simulink model "sim_tcyb_2024_att_ctrl"  (R2020a)
settings: Solver=ode4  StartTime=0.0  StopTime=30.0  FixedStep=0.01  RelTol=1e-3
values from neighbouring files (symbols this model uses):
  c1_diff_sigma_bar_w = diag([12; 12; 12])    [init_tcyb_2024_att_ctrl.m]
  c1_diff_ui = diag([25; 30; 20])    [init_tcyb_2024_att_ctrl.m]
  c2_diff_sigma_bar_w = diag([12; 12; 12])    [init_tcyb_2024_att_ctrl.m]
  c2_diff_ui = diag([50; 50; 10])    [init_tcyb_2024_att_ctrl.m]
  c3_diff_sigma_bar_w = diag([15; 15; 15])    [init_tcyb_2024_att_ctrl.m]
  c3_diff_ui = diag([15; 15; 10])    [init_tcyb_2024_att_ctrl.m]
  dw_aa_t = 0.2 * ones(3, 5) + ( 1.0 - 0.2 ) * rand(3, 5)    [init_tcyb_2024_att_ctrl.m]
  dw_ff_t = [ 0.4 * ones(1, 5) + ( 1.0 - 0.4 ) * rand(1, 5);                      0.4 * ones(1, 5) + ( 1.0 - 0.4 ) * rand(1, 5);                      0.2 * ones(1, 5) + ( 0.6 - 0.2 ) * rand(1, 5) ]    [init_tcyb_2024_att_ctrl.m]
  dw_phi_t = ( - pi / 2 ) * ones(3, 5) + ( pi / 2 - ( - pi / 2 ) ) * rand(3, 5)    [init_tcyb_2024_att_ctrl.m]
  dwci_init = zeros(3,NF)    [init_tcyb_2024_att_ctrl.m]
  h1w = diag([20.0; 20.0; 20.0])    [init_tcyb_2024_att_ctrl.m]
  h2w = diag([30.0; 35.0; 35.0])    [init_tcyb_2024_att_ctrl.m]
  h3w = diag([30.0; 25.0; 30.0])    [init_tcyb_2024_att_ctrl.m]
  Ji = zeros(3,3,NF)    [init_tcyb_2024_att_ctrl.m]
  ksg = diag([10.0, 10.0, 8.0])    [init_tcyb_2024_att_ctrl.m]
  kw = diag([10.0, 10.0, 8.0])    [init_tcyb_2024_att_ctrl.m]
  l1 = diag([5.0, 5.0, 4.0])    [init_tcyb_2024_att_ctrl.m]
  l2 = diag([5.0, 5.0, 4.0])    [init_tcyb_2024_att_ctrl.m]
  Lamd_diff_sigma_bar_w = 0.8    [init_tcyb_2024_att_ctrl.m]
  Lamd_diff_ui = 0.8    [init_tcyb_2024_att_ctrl.m]
  mu = diag([10.0, 10.0, 10.0, 8.0, 8.0, 8.0])    [init_tcyb_2024_att_ctrl.m]
  mu_d_w = 100    [init_tcyb_2024_att_ctrl.m]
  pos0 = zeros(3, 1)    [init_tcyb_2024_att_ctrl.m]
  PZ0 = P0(3)    [init_tcyb_2024_att_ctrl.m]
  PZ1 = 10    [init_tcyb_2024_att_ctrl.m]
  R0 = 4    [init_tcyb_2024_att_ctrl.m]
  R1 = 8    [init_tcyb_2024_att_ctrl.m]
  Rei_init = zeros(3,3,NF)    [init_tcyb_2024_att_ctrl.m]
  Ri_init = zeros(3,3,NF)    [init_tcyb_2024_att_ctrl.m]
  Rx2 = 10    [init_tcyb_2024_att_ctrl.m]
  Ry2 = 6    [init_tcyb_2024_att_ctrl.m]
  Rz2 = 4    [init_tcyb_2024_att_ctrl.m]
  sgei_init = zeros(3,NF)    [init_tcyb_2024_att_ctrl.m]
  sgi_init = zeros(3,NF)    [init_tcyb_2024_att_ctrl.m]
  T0 = 0    [init_tcyb_2024_att_ctrl.m]
  T1 = tseq1    (= 10)    [init_tcyb_2024_att_ctrl.m]
  T2 = tseq1 + tseq12 + tseq2    (= 30)    [init_tcyb_2024_att_ctrl.m]
  ui_init = zeros(3,NF)    [init_tcyb_2024_att_ctrl.m]
  V_Phi_Rei_init = zeros(3,NF)    [init_tcyb_2024_att_ctrl.m]
  vel0 = zeros(3, 1)    [init_tcyb_2024_att_ctrl.m]
  wci_init = zeros(3,NF)    [init_tcyb_2024_att_ctrl.m]
  wei_init = zeros(3,NF)    [init_tcyb_2024_att_ctrl.m]
  zeta_diff_sigma_bar_w = 0.3    [init_tcyb_2024_att_ctrl.m]
  zeta_diff_ui = 0.05    [init_tcyb_2024_att_ctrl.m]
undefined symbols (not defined in the file or in its folder): cal_frac_squ, p_alfaw1, p_alfaw2, q_alfaw1, q_alfaw2, wi_init
(part 4 of 5)

== matlab function sim_tcyb_2024_att_ctrl/combine wei Qei Rei ==
  data: wei_1 input; wei_vec output; wei_2 input; wei_3 input; wei_4 input; wei_5 input; sgei_1 input; sgei_2 input; sgei_3 input; sgei_4 input; sgei_5 input; Rei_1 input; Rei_2 input; Rei_3 input; Rei_4 input; Rei_5 input; sgei_vec output; Rei_vec output
function [wei_vec, sgei_vec, Rei_vec] = fcn(wei_1, wei_2, wei_3, wei_4, wei_5, ...
                                                                                sgei_1, sgei_2, sgei_3, sgei_4, sgei_5, ...
                                                                                Rei_1, Rei_2, Rei_3, Rei_4, Rei_5)
%%%% 合并姿态角速率误差/四元数误差/姿态旋转矩阵误差
wei_vec = zeros(3,5);
wei_vec(:,1) = wei_1(:);
wei_vec(:,2) = wei_2(:);
wei_vec(:,3) = wei_3(:);
wei_vec(:,4) = wei_4(:);
wei_vec(:,5) = wei_5(:);

sgei_vec = zeros(3,5);
sgei_vec(:,1) = sgei_1(:);
sgei_vec(:,2) = sgei_2(:);
sgei_vec(:,3) = sgei_3(:);
sgei_vec(:,4) = sgei_4(:);
sgei_vec(:,5) = sgei_5(:);

Rei_vec = zeros(3,3,5);
Rei_vec(:,:,1) = Rei_1;
Rei_vec(:,:,2) = Rei_2;
Rei_vec(:,:,3) = Rei_3;
Rei_vec(:,:,4) = Rei_4;
Rei_vec(:,:,5) = Rei_5;

== matlab function sim_tcyb_2024_att_ctrl/cal Ri agent 1 ==
  data: Ri_1 output; sgi_vec input
function Ri_1 = fcn(sgi_vec)
%%%% 由罗德里格常量sgi求解姿态旋转矩阵Ri
iiuav = 1;
Ri_1 = eye(3) + 4 * ( 1 - ( ( ( sgi_vec(:,iiuav)' ) * sgi_vec(:,iiuav) ) / ( ( 1 + ( sgi_vec(:,iiuav)' ) * sgi_vec(:,iiuav) ) ^ 2 ) ) ) * cal_askew_mat( sgi_vec(:,iiuav) ) ...
                            + ( 8 / ( ( 1 + ( sgi_vec(:,iiuav)' ) * sgi_vec(:,iiuav) ) ^ 2 ) ) * cal_askew_mat( sgi_vec(:,iiuav) ) * cal_askew_mat( sgi_vec(:,iiuav) );
Ri_1 = Ri_1';
end

== matlab function sim_tcyb_2024_att_ctrl/combine E_sgi_vec ==
  data: E_sgi_1 input; E_sgi_vec output; E_sgi_2 input; E_sgi_3 input; E_sgi_4 input; E_sgi_5 input
function E_sgi_vec = fcn(E_sgi_1, E_sgi_2, E_sgi_3, E_sgi_4, E_sgi_5)
%%%% 合并姿态计算矩阵
E_sgi_vec = zeros(3,3,5);
E_sgi_vec(:,:,1) = E_sgi_1;
E_sgi_vec(:,:,2) = E_sgi_2;
E_sgi_vec(:,:,3) = E_sgi_3;
E_sgi_vec(:,:,4) = E_sgi_4;
E_sgi_vec(:,:,5) = E_sgi_5;

== matlab function sim_tcyb_2024_att_ctrl/cal differentiator d_sigma_bar_w_hat agent 3/choose sigma_bar_w ==
  data: x input; y output
function y = fcn(x)
iiuav = 3;
y = x(:,iiuav);

== matlab function sim_tcyb_2024_att_ctrl/cal differentiator d_sigma_bar_w_hat agent 3/trans to column20 ==
  data: x input; y output
function y = fcn(x)
y = x(:);

== matlab function sim_tcyb_2024_att_ctrl/cal differentiator d_sigma_bar_w_hat agent 3/trans to column21 ==
  data: x input; y output
function y = fcn(x)
y = x(:);

== matlab function sim_tcyb_2024_att_ctrl/cal differentiator d_sigma_bar_w_hat agent 3/trans to column22 ==
  data: x input; y output
function y = fcn(x)
y = x(:);

== matlab function sim_tcyb_2024_att_ctrl/cal differentiator d_sigma_bar_w_hat agent 3/trans to column23 ==
  data: x input; y output
function y = fcn(x)
y = x(:);

== matlab function sim_tcyb_2024_att_ctrl/combine Qci Rci1 ==
  data: V_Phi_Rei_1 input; V_Phi_Rei_vec output; V_Phi_Rei_2 input; V_Phi_Rei_3 input; V_Phi_Rei_4 input; V_Phi_Rei_5 input
function V_Phi_Rei_vec = fcn(V_Phi_Rei_1, V_Phi_Rei_2, V_Phi_Rei_3, V_Phi_Rei_4, V_Phi_Rei_5)
%%%% 合并LogSO3空间的辅助姿态误差向量
V_Phi_Rei_vec = [V_Phi_Rei_1(:), V_Phi_Rei_2(:), V_Phi_Rei_3(:), V_Phi_Rei_4(:), V_Phi_Rei_5(:)];

== matlab function sim_tcyb_2024_att_ctrl/depart sge1 ==
  data: y output; x input
function y = fcn(x)
y = x(:,1);

end

== matlab function sim_tcyb_2024_att_ctrl/depart sge2 ==
  data: y output; x input
function y = fcn(x)
y = x(:,2);

end

== matlab function sim_tcyb_2024_att_ctrl/depart sge3 ==
  data: y output; x input
function y = fcn(x)
y = x(:,3);

end

== matlab function sim_tcyb_2024_att_ctrl/depart sge4 ==
  data: y output; x input
function y = fcn(x)
y = x(:,4);

end

== matlab function sim_tcyb_2024_att_ctrl/depart sge5 ==
  data: y output; x input
function y = fcn(x)
y = x(:,5);

end

== matlab function sim_tcyb_2024_att_ctrl/depart we1 ==
  data: y output; x input
function y = fcn(x)
y = x(:,1);

end

== matlab function sim_tcyb_2024_att_ctrl/depart we2 ==
  data: y output; x input
function y = fcn(x)
y = x(:,2);

end

== matlab function sim_tcyb_2024_att_ctrl/depart we3 ==
  data: y output; x input
function y = fcn(x)
y = x(:,3);

end

== matlab function sim_tcyb_2024_att_ctrl/depart we4 ==
  data: y output; x input
function y = fcn(x)
y = x(:,4);

end

== matlab function sim_tcyb_2024_att_ctrl/E_sgi agent 3 ==
  data: sgi_vec input; E_sgi_3 output
function E_sgi_3 = fcn(sgi_vec)
%%%% 更新四元数微分方程
iiuav = 3;
E_sgi_3 = (1/4) * ( ( 1 - (sgi_vec(:,iiuav)') * sgi_vec(:,iiuav) ) * eye(3) ...
                    + 2 * cal_askew_mat( sgi_vec(:,iiuav) ) + 2 * sgi_vec(:,iiuav) * ( sgi_vec(:,iiuav)' ) );
end

== matlab function sim_tcyb_2024_att_ctrl/depart we5 ==
  data: y output; x input
function y = fcn(x)
y = x(:,5);

end

== matlab function sim_tcyb_2024_att_ctrl/depart V_Phi_Re5 ==
  data: y output; x input
function y = fcn(x)
y = x(:,5);

end

== matlab function sim_tcyb_2024_att_ctrl/depart V_Phi_Re1 ==
  data: y output; x input
function y = fcn(x)
y = x(:,1);

end

== matlab function sim_tcyb_2024_att_ctrl/depart V_Phi_Re2 ==
  data: y output; x input
function y = fcn(x)
y = x(:,2);

end

== matlab function sim_tcyb_2024_att_ctrl/depart V_Phi_Re3 ==
  data: y output; x input
function y = fcn(x)
y = x(:,3);

end

== matlab function sim_tcyb_2024_att_ctrl/depart V_Phi_Re4 ==
  data: y output; x input
function y = fcn(x)
y = x(:,4);

end

== matlab function sim_tcyb_2024_att_ctrl/cal differentiator d_sigma_bar_w_hat agent 3/trans to column24 ==
  data: x input; y output
function y = fcn(x)
y = x(:);

== matlab function sim_tcyb_2024_att_ctrl/cal differentiator d_sigma_bar_w_hat agent 3/trans to column25 ==
  data: x input; y output
function y = fcn(x)
y = x(:);

== matlab function sim_tcyb_2024_att_ctrl/cal differentiator d_sigma_bar_w_hat agent 4/cal differentiator ==
  data: c1 input; d_sigma_bar_v_hat output; d_dsigma_bar_v_hat output; d_d2sigma_bar_v_hat output; c2 input; c3 input; chi_t input; sigma_bar_v_sig_1 input; sigma_bar_v_sig_2 input; sigma_bar_v_sig_3 input; sigma_bar_v_sig_4 input; sigma_bar_v_sig_5 input; sigma_bar_v_sig_6 input; d_sigma_bar_v_hat input; d2_sigma_bar_v_hat input
function [d_sigma_bar_v_hat, d_dsigma_bar_v_hat, d_d2sigma_bar_v_hat] = fcn(c1, c2, c3, chi_t, sigma_bar_v_sig_1, sigma_bar_v_sig_2, sigma_bar_v_sig_3, ...
                                                                                                                                                sigma_bar_v_sig_4, sigma_bar_v_sig_5, sigma_bar_v_sig_6, d_sigma_bar_v_hat, d2_sigma_bar_v_hat)
d_d2sigma_bar_v_hat = -chi_t .* c1 * sigma_bar_v_sig_1(:) - (1 - chi_t) .* c1 * sigma_bar_v_sig_2(:);
d_dsigma_bar_v_hat = -chi_t .* c2 * sigma_bar_v_sig_3(:) - (1 - chi_t) .* c2 * sigma_bar_v_sig_4(:) + d2_sigma_bar_v_hat(:);
d_sigma_bar_v_hat = -chi_t .* c3 * sigma_bar_v_sig_5(:) - (1 - chi_t) .* c3 * sigma_bar_v_sig_6(:) + d_sigma_bar_v_hat(:);

== matlab function sim_tcyb_2024_att_ctrl/sgi dynam agent 3 ==
  data: E_sgi_vec input; dsgi_3 output; wi_vec input
function dsgi_3 = fcn(E_sgi_vec, wi_vec)
%%%% 更新四元数微分方程
iiuav = 3;
dsgi_3 = E_sgi_vec(:,:,iiuav) * wi_vec(:,iiuav);
end

== matlab function sim_tcyb_2024_att_ctrl/cal differentiator d_sigma_bar_w_hat agent 4/cal sig ==
  data: x input; z output; y input
function z = fcn(x, y)
z = x(:) .* sign(y(:));

== matlab function sim_tcyb_2024_att_ctrl/cal differentiator d_sigma_bar_w_hat agent 4/cal sig1 ==
  data: x input; z output; y input
function z = fcn(x, y)
z = x(:) .* sign(y(:));

== matlab function sim_tcyb_2024_att_ctrl/cal differentiator d_sigma_bar_w_hat agent 4/cal sig2 ==
  data: x input; z output; y input
function z = fcn(x, y)
z = x(:) .* sign(y(:));

== matlab function sim_tcyb_2024_att_ctrl/cal differentiator d_sigma_bar_w_hat agent 4/cal sig3 ==
  data: x input; z output; y input
function z = fcn(x, y)
z = x(:) .* sign(y(:));

== matlab function sim_tcyb_2024_att_ctrl/cal differentiator d_sigma_bar_w_hat agent 4/cal sig4 ==
  data: x input; z output; y input
function z = fcn(x, y)
z = x(:) .* sign(y(:));

== matlab function sim_tcyb_2024_att_ctrl/cal differentiator d_sigma_bar_w_hat agent 4/cal sig5 ==
  data: x input; z output; y input
function z = fcn(x, y)
z = x(:) .* sign(y(:));

== matlab function sim_tcyb_2024_att_ctrl/cal differentiator d_sigma_bar_w_hat agent 4/choose sigma_bar_w ==
  data: x input; y output
function y = fcn(x)
iiuav = 4;
y = x(:,iiuav);

== matlab function sim_tcyb_2024_att_ctrl/cal differentiator d_sigma_bar_w_hat agent 4/trans to column20 ==
  data: x input; y output
function y = fcn(x)
y = x(:);

== matlab function sim_tcyb_2024_att_ctrl/cal differentiator d_sigma_bar_w_hat agent 4/trans to column21 ==
  data: x input; y output
function y = fcn(x)
y = x(:);

== matlab function sim_tcyb_2024_att_ctrl/cal differentiator d_sigma_bar_w_hat agent 4/trans to column22 ==
  data: x input; y output
function y = fcn(x)
y = x(:);

== matlab function sim_tcyb_2024_att_ctrl/cal Ri agent 4 ==
  data: Ri_4 output; sgi_vec input
function Ri_4 = fcn(sgi_vec)
%%%% 由罗德里格常量sgi求解姿态旋转矩阵Ri
iiuav = 4;
Ri_4 = eye(3) + 4 * ( 1 - ( ( ( sgi_vec(:,iiuav)' ) * sgi_vec(:,iiuav) ) / ( ( 1 + ( sgi_vec(:,iiuav)' ) * sgi_vec(:,iiuav) ) ^ 2 ) ) ) * cal_askew_mat( sgi_vec(:,iiuav) ) ...
                            + ( 8 / ( ( 1 + ( sgi_vec(:,iiuav)' ) * sgi_vec(:,iiuav) ) ^ 2 ) ) * cal_askew_mat( sgi_vec(:,iiuav) ) * cal_askew_mat( sgi_vec(:,iiuav) );
Ri_4 = Ri_4';
end

== matlab function sim_tcyb_2024_att_ctrl/cal differentiator d_sigma_bar_w_hat agent 4/trans to column23 ==
  data: x input; y output
function y = fcn(x)
y = x(:);

== matlab function sim_tcyb_2024_att_ctrl/cal differentiator d_sigma_bar_w_hat agent 4/trans to column24 ==
  data: x input; y output
function y = fcn(x)
y = x(:);

== matlab function sim_tcyb_2024_att_ctrl/cal differentiator d_sigma_bar_w_hat agent 4/trans to column25 ==
  data: x input; y output
function y = fcn(x)
y = x(:);

== matlab function sim_tcyb_2024_att_ctrl/cal differentiator d_sigma_bar_w_hat agent 5/cal differentiator ==
  data: c1 input; d_sigma_bar_v_hat output; d_dsigma_bar_v_hat output; d_d2sigma_bar_v_hat output; c2 input; c3 input; chi_t input; sigma_bar_v_sig_1 input; sigma_bar_v_sig_2 input; sigma_bar_v_sig_3 input; sigma_bar_v_sig_4 input; sigma_bar_v_sig_5 input; sigma_bar_v_sig_6 input; d_sigma_bar_v_hat input; d2_sigma_bar_v_hat input
function [d_sigma_bar_v_hat, d_dsigma_bar_v_hat, d_d2sigma_bar_v_hat] = fcn(c1, c2, c3, chi_t, sigma_bar_v_sig_1, sigma_bar_v_sig_2, sigma_bar_v_sig_3, ...
                                                                                                                                                sigma_bar_v_sig_4, sigma_bar_v_sig_5, sigma_bar_v_sig_6, d_sigma_bar_v_hat, d2_sigma_bar_v_hat)
d_d2sigma_bar_v_hat = -chi_t .* c1 * sigma_bar_v_sig_1(:) - (1 - chi_t) .* c1 * sigma_bar_v_sig_2(:);
d_dsigma_bar_v_hat = -chi_t .* c2 * sigma_bar_v_sig_3(:) - (1 - chi_t) .* c2 * sigma_bar_v_sig_4(:) + d2_sigma_bar_v_hat(:);
d_sigma_bar_v_hat = -chi_t .* c3 * sigma_bar_v_sig_5(:) - (1 - chi_t) .* c3 * sigma_bar_v_sig_6(:) + d_sigma_bar_v_hat(:);

== matlab function sim_tcyb_2024_att_ctrl/cal differentiator d_sigma_bar_w_hat agent 5/cal sig ==
  data: x input; z output; y input
function z = fcn(x, y)
z = x(:) .* sign(y(:));

== matlab function sim_tcyb_2024_att_ctrl/cal differentiator d_sigma_bar_w_hat agent 5/cal sig1 ==
  data: x input; z output; y input
function z = fcn(x, y)
z = x(:) .* sign(y(:));

== matlab function sim_tcyb_2024_att_ctrl/cal differentiator d_sigma_bar_w_hat agent 5/cal sig2 ==
  data: x input; z output; y input
function z = fcn(x, y)
z = x(:) .* sign(y(:));

== matlab function sim_tcyb_2024_att_ctrl/E_sgi agent 4 ==
  data: sgi_vec input; E_sgi_4 output
function E_sgi_4 = fcn(sgi_vec)
%%%% 更新四元数微分方程
iiuav = 4;
E_sgi_4 = (1/4) * ( ( 1 - (sgi_vec(:,iiuav)') * sgi_vec(:,iiuav) ) * eye(3) ...
                    + 2 * cal_askew_mat( sgi_vec(:,iiuav) ) + 2 * sgi_vec(:,iiuav) * ( sgi_vec(:,iiuav)' ) );
end

== matlab function sim_tcyb_2024_att_ctrl/cal differentiator d_sigma_bar_w_hat agent 5/cal sig3 ==
  data: x input; z output; y input
function z = fcn(x, y)
z = x(:) .* sign(y(:));

== matlab function sim_tcyb_2024_att_ctrl/cal differentiator d_sigma_bar_w_hat agent 5/cal sig4 ==
  data: x input; z output; y input
function z = fcn(x, y)
z = x(:) .* sign(y(:));

== matlab function sim_tcyb_2024_att_ctrl/cal differentiator d_sigma_bar_w_hat agent 5/cal sig5 ==
  data: x input; z output; y input
function z = fcn(x, y)
z = x(:) .* sign(y(:));

== matlab function sim_tcyb_2024_att_ctrl/cal differentiator d_sigma_bar_w_hat agent 5/choose sigma_bar_w ==
  data: x input; y output
function y = fcn(x)
iiuav = 5;
y = x(:,iiuav);

== matlab function sim_tcyb_2024_att_ctrl/cal differentiator d_sigma_bar_w_hat agent 5/trans to column20 ==
  data: x input; y output
function y = fcn(x)
y = x(:);

== matlab function sim_tcyb_2024_att_ctrl/cal differentiator d_sigma_bar_w_hat agent 5/trans to column21 ==
  data: x input; y output
function y = fcn(x)
y = x(:);

== matlab function sim_tcyb_2024_att_ctrl/cal differentiator d_sigma_bar_w_hat agent 5/trans to column22 ==
  data: x input; y output
function y = fcn(x)
y = x(:);

== matlab function sim_tcyb_2024_att_ctrl/cal differentiator d_sigma_bar_w_hat agent 5/trans to column23 ==
  data: x input; y output
function y = fcn(x)
y = x(:);

== matlab function sim_tcyb_2024_att_ctrl/cal differentiator d_sigma_bar_w_hat agent 5/trans to column24 ==
  data: x input; y output
function y = fcn(x)
y = x(:);

== matlab function sim_tcyb_2024_att_ctrl/cal differentiator d_sigma_bar_w_hat agent 5/trans to column25 ==
  data: x input; y output
function y = fcn(x)
y = x(:);

== matlab function sim_tcyb_2024_att_ctrl/sgi dynam agent 4 ==
  data: E_sgi_vec input; dsgi_4 output; wi_vec input
function dsgi_4 = fcn(E_sgi_vec, wi_vec)
%%%% 更新四元数微分方程
iiuav = 4;
dsgi_4 = E_sgi_vec(:,:,iiuav) * wi_vec(:,iiuav);
end

== matlab function sim_tcyb_2024_att_ctrl/cal dw_hat agent 1 ==
  data: h3w input; Ji input; d_sigma_bar_w_vec input; sigma_bar_w_hat_vec input; dw_hat_1 output
function dw_hat_1 = fcn(h3w, Ji, d_sigma_bar_w_vec, sigma_bar_w_hat_vec)
%%%% 计算扰动观测值dw_hat
iiuav = 1;
dw_hat_1 = Ji(:,:,iiuav) * d_sigma_bar_w_vec(:,iiuav) + h3w * sigma_bar_w_hat_vec(:,iiuav);

== matlab function sim_tcyb_2024_att_ctrl/cal dw_hat agent 2 ==
  data: h3w input; Ji input; d_sigma_bar_w_vec input; sigma_bar_w_hat_vec input; dw_hat_2 output
function dw_hat_2 = fcn(h3w, Ji, d_sigma_bar_w_vec, sigma_bar_w_hat_vec)
%%%% 计算扰动观测值dw_hat
iiuav = 2;
dw_hat_2 = Ji(:,:,iiuav) * d_sigma_bar_w_vec(:,iiuav) + h3w * sigma_bar_w_hat_vec(:,iiuav);

== matlab function sim_tcyb_2024_att_ctrl/cal dw_hat agent 3 ==
  data: h3w input; Ji input; d_sigma_bar_w_vec input; sigma_bar_w_hat_vec input; dw_hat_3 output
function dw_hat_3 = fcn(h3w, Ji, d_sigma_bar_w_vec, sigma_bar_w_hat_vec)
%%%% 计算扰动观测值dw_hat
iiuav = 3;
dw_hat_3 = Ji(:,:,iiuav) * d_sigma_bar_w_vec(:,iiuav) + h3w * sigma_bar_w_hat_vec(:,iiuav);

== matlab function sim_tcyb_2024_att_ctrl/cal dw_hat agent 4 ==
  data: h3w input; Ji input; d_sigma_bar_w_vec input; sigma_bar_w_hat_vec input; dw_hat_4 output
function dw_hat_4 = fcn(h3w, Ji, d_sigma_bar_w_vec, sigma_bar_w_hat_vec)
%%%% 计算扰动观测值dw_hat
iiuav = 4;
dw_hat_4 = Ji(:,:,iiuav) * d_sigma_bar_w_vec(:,iiuav) + h3w * sigma_bar_w_hat_vec(:,iiuav);

== matlab function sim_tcyb_2024_att_ctrl/cal dw_hat agent 5 ==
  data: h3w input; Ji input; d_sigma_bar_w_vec input; sigma_bar_w_hat_vec input; dw_hat_5 output
function dw_hat_5 = fcn(h3w, Ji, d_sigma_bar_w_vec, sigma_bar_w_hat_vec)
%%%% 计算扰动观测值dw_hat
iiuav = 5;
dw_hat_5 = Ji(:,:,iiuav) * d_sigma_bar_w_vec(:,iiuav) + h3w * sigma_bar_w_hat_vec(:,iiuav);

== matlab function sim_tcyb_2024_att_ctrl/cal error dw_tilt ==
  data: dw_vec input; dw_hat_vec input; dw_tilt_vec output
function dw_tilt_vec = fcn(dw_vec, dw_hat_vec)
%%%% 计算扰动观测误差dw_tilt
dw_tilt_vec = zeros(3,5);
for iiuav = 1:5
    dw_tilt_vec(:,iiuav) = dw_vec(:,iiuav) - dw_hat_vec(:,iiuav);
end

== matlab function sim_tcyb_2024_att_ctrl/cal sigma_bar_w_hat agent 1 ==
  data: h1w input; h2w input; theta_sigma_bar_w_tilt_1_vec input; d_sigma_bar_w_hat_1 output; theta_sigma_bar_w_tilt_2_vec input; d_sigma_bar_w_vec input
function d_sigma_bar_w_hat_1 = fcn(h1w, h2w, theta_sigma_bar_w_tilt_1_vec, theta_sigma_bar_w_tilt_2_vec, d_sigma_bar_w_vec)
%%%% 计算扰动观测器中虚拟速度控制量观测值sigma_w_hat的微分方程
iiuav = 1;
d_sigma_bar_w_hat_1 = d_sigma_bar_w_vec(:,iiuav) + ...
                                            h1w * theta_sigma_bar_w_tilt_1_vec(:,iiuav) + ...
                                            h2w * theta_sigma_bar_w_tilt_2_vec(:,iiuav);

== matlab function sim_tcyb_2024_att_ctrl/cal sigma_bar_w_hat agent 2 ==
  data: h1w input; h2w input; theta_sigma_bar_w_tilt_1_vec input; d_sigma_bar_w_hat_2 output; theta_sigma_bar_w_tilt_2_vec input; d_sigma_bar_w_vec input
function d_sigma_bar_w_hat_2 = fcn(h1w, h2w, theta_sigma_bar_w_tilt_1_vec, theta_sigma_bar_w_tilt_2_vec, d_sigma_bar_w_vec)
%%%% 计算扰动观测器中虚拟速度控制量观测值sigma_v_hat的微分方程
iiuav = 2;
d_sigma_bar_w_hat_2 = d_sigma_bar_w_vec(:,iiuav) + ...
                                            h1w * theta_sigma_bar_w_tilt_1_vec(:,iiuav) + ...
                                            h2w * theta_sigma_bar_w_tilt_2_vec(:,iiuav);

== matlab function sim_tcyb_2024_att_ctrl/cal Ri agent 5 ==
  data: Ri_5 output; sgi_vec input
function Ri_5 = fcn(sgi_vec)
%%%% 由罗德里格常量sgi求解姿态旋转矩阵Ri
iiuav = 5;
Ri_5 = eye(3) + 4 * ( 1 - ( ( ( sgi_vec(:,iiuav)' ) * sgi_vec(:,iiuav) ) / ( ( 1 + ( sgi_vec(:,iiuav)' ) * sgi_vec(:,iiuav) ) ^ 2 ) ) ) * cal_askew_mat( sgi_vec(:,iiuav) ) ...
                            + ( 8 / ( ( 1 + ( sgi_vec(:,iiuav)' ) * sgi_vec(:,iiuav) ) ^ 2 ) ) * cal_askew_mat( sgi_vec(:,iiuav) ) * cal_askew_mat( sgi_vec(:,iiuav) );
Ri_5 = Ri_5';
end

== matlab function sim_tcyb_2024_att_ctrl/cal sigma_bar_w_hat agent 3 ==
  data: h1w input; h2w input; theta_sigma_bar_w_tilt_1_vec input; d_sigma_bar_w_hat_3 output; theta_sigma_bar_w_tilt_2_vec input; d_sigma_bar_w_vec input
function d_sigma_bar_w_hat_3 = fcn(h1w, h2w, theta_sigma_bar_w_tilt_1_vec, theta_sigma_bar_w_tilt_2_vec, d_sigma_bar_w_vec)
%%%% 计算扰动观测器中虚拟速度控制量观测值sigma_w_hat的微分方程
iiuav = 3;
d_sigma_bar_w_hat_3 = d_sigma_bar_w_vec(:,iiuav) + ...
                                            h1w * theta_sigma_bar_w_tilt_1_vec(:,iiuav) + ...
                                            h2w * theta_sigma_bar_w_tilt_2_vec(:,iiuav);

== matlab function sim_tcyb_2024_att_ctrl/cal sigma_bar_w_hat agent 4 ==
  data: h1w input; h2w input; theta_sigma_bar_w_tilt_1_vec input; d_sigma_bar_w_hat_4 output; theta_sigma_bar_w_tilt_2_vec input; d_sigma_bar_w_vec input
function d_sigma_bar_w_hat_4 = fcn(h1w, h2w, theta_sigma_bar_w_tilt_1_vec, theta_sigma_bar_w_tilt_2_vec, d_sigma_bar_w_vec)
%%%% 计算扰动观测器中虚拟速度控制量观测值sigma_w_hat的微分方程
iiuav = 4;
d_sigma_bar_w_hat_4 = d_sigma_bar_w_vec(:,iiuav) + ...
                                            h1w * theta_sigma_bar_w_tilt_1_vec(:,iiuav) + ...
                                            h2w * theta_sigma_bar_w_tilt_2_vec(:,iiuav);

== matlab function sim_tcyb_2024_att_ctrl/cal sigma_bar_w_hat agent 5 ==
  data: h1w input; h2w input; theta_sigma_bar_w_tilt_1_vec input; d_sigma_bar_w_hat_5 output; theta_sigma_bar_w_tilt_2_vec input; d_sigma_bar_w_vec input
function d_sigma_bar_w_hat_5 = fcn(h1w, h2w, theta_sigma_bar_w_tilt_1_vec, theta_sigma_bar_w_tilt_2_vec, d_sigma_bar_w_vec)
%%%% 计算扰动观测器中虚拟速度控制量观测值sigma_w_hat的微分方程
iiuav = 5;
d_sigma_bar_w_hat_5 = d_sigma_bar_w_vec(:,iiuav) + ...
                                            h1w * theta_sigma_bar_w_tilt_1_vec(:,iiuav) + ...
                                            h2w * theta_sigma_bar_w_tilt_2_vec(:,iiuav);

== matlab function sim_tcyb_2024_att_ctrl/cal sigma_w_bar ==
  data: sigma_bar_w_vec output; wi_vec input; sigma_w_vec input
function sigma_bar_w_vec = fcn(wi_vec, sigma_w_vec)
%%%% 计算姿态角速率跟踪误差
sigma_bar_w_vec = zeros(3,5);
for iiuav = 1:5
    sigma_bar_w_vec(:,iiuav) = wi_vec(:,iiuav) - sigma_w_vec(:,iiuav);
end

== matlab function sim_tcyb_2024_att_ctrl/cal theta_sigma_bar_w_tilt agent 1 ==
  data: alfa_theta_obs_w input; sigma_bar_w_tilt_squ_1_1 input; theta_sigma_bar_w_tilt_1_1 output; sigma_bar_w_tilt_squ_2_1 input; sigma_bar_w_tilt_vec input; theta_sigma_bar_w_tilt_2_1 output
function [theta_sigma_bar_w_tilt_1_1, theta_sigma_bar_w_tilt_2_1] = fcn(alfa_theta_obs_w, sigma_bar_w_tilt_squ_1_1, sigma_bar_w_tilt_squ_2_1, sigma_bar_w_tilt_vec)
%%%% 计算平滑递增函数
iiuav = 1;
theta_sigma_bar_w_tilt_1_1 = sigma_bar_w_tilt_squ_1_1(:) .* ( -1 + 2 ./ ( 1 + exp( -alfa_theta_obs_w .* sigma_bar_w_tilt_vec(:,iiuav) ) ) );
theta_sigma_bar_w_tilt_2_1 = sigma_bar_w_tilt_squ_2_1(:) .* ( -1 + 2 ./ ( 1 + exp( -alfa_theta_obs_w .* sigma_bar_w_tilt_vec(:,iiuav) ) ) );

== matlab function sim_tcyb_2024_att_ctrl/cal theta_sigma_bar_w_tilt agent 2 ==
  data: alfa_theta_obs_w input; sigma_bar_w_tilt_squ_1_2 input; theta_sigma_bar_w_tilt_1_2 output; sigma_bar_w_tilt_squ_2_2 input; sigma_bar_w_tilt_vec input; theta_sigma_bar_w_tilt_2_2 output
function [theta_sigma_bar_w_tilt_1_2, theta_sigma_bar_w_tilt_2_2] = fcn(alfa_theta_obs_w, sigma_bar_w_tilt_squ_1_2, sigma_bar_w_tilt_squ_2_2, sigma_bar_w_tilt_vec)
%%%% 计算平滑递增函数
iiuav = 2;
theta_sigma_bar_w_tilt_1_2 = sigma_bar_w_tilt_squ_1_2(:) .* ( -1 + 2 ./ ( 1 + exp( -alfa_theta_obs_w .* sigma_bar_w_tilt_vec(:,iiuav) ) ) );
theta_sigma_bar_w_tilt_2_2 = sigma_bar_w_tilt_squ_2_2(:) .* ( -1 + 2 ./ ( 1 + exp( -alfa_theta_obs_w .* sigma_bar_w_tilt_vec(:,iiuav) ) ) );

== matlab function sim_tcyb_2024_att_ctrl/cal theta_sigma_bar_w_tilt agent 3 ==
  data: alfa_theta_obs_w input; sigma_bar_w_tilt_squ_1_3 input; theta_sigma_bar_w_tilt_1_3 output; sigma_bar_w_tilt_squ_2_3 input; sigma_bar_w_tilt_vec input; theta_sigma_bar_w_tilt_2_3 output
function [theta_sigma_bar_w_tilt_1_3, theta_sigma_bar_w_tilt_2_3] = fcn(alfa_theta_obs_w, sigma_bar_w_tilt_squ_1_3, sigma_bar_w_tilt_squ_2_3, sigma_bar_w_tilt_vec)
%%%% 计算平滑递增函数
iiuav = 3;
theta_sigma_bar_w_tilt_1_3 = sigma_bar_w_tilt_squ_1_3(:) .* ( -1 + 2 ./ ( 1 + exp( -alfa_theta_obs_w .* sigma_bar_w_tilt_vec(:,iiuav) ) ) );
theta_sigma_bar_w_tilt_2_3 = sigma_bar_w_tilt_squ_2_3(:) .* ( -1 + 2 ./ ( 1 + exp( -alfa_theta_obs_w .* sigma_bar_w_tilt_vec(:,iiuav) ) ) );

== matlab function sim_tcyb_2024_att_ctrl/E_sgi agent 5 ==
  data: sgi_vec input; E_sgi_5 output
function E_sgi_5 = fcn(sgi_vec)
%%%% 更新四元数微分方程
iiuav = 5;
E_sgi_5 = (1/4) * ( ( 1 - (sgi_vec(:,iiuav)') * sgi_vec(:,iiuav) ) * eye(3) ...
                    + 2 * cal_askew_mat( sgi_vec(:,iiuav) ) + 2 * sgi_vec(:,iiuav) * ( sgi_vec(:,iiuav)' ) );
end

== matlab function sim_tcyb_2024_att_ctrl/cal theta_sigma_bar_w_tilt agent 4 ==
  data: alfa_theta_obs_w input; sigma_bar_w_tilt_squ_1_4 input; theta_sigma_bar_w_tilt_1_4 output; sigma_bar_w_tilt_squ_2_4 input; sigma_bar_w_tilt_vec input; theta_sigma_bar_w_tilt_2_4 output
function [theta_sigma_bar_w_tilt_1_4, theta_sigma_bar_w_tilt_2_4] = fcn(alfa_theta_obs_w, sigma_bar_w_tilt_squ_1_4, sigma_bar_w_tilt_squ_2_4, sigma_bar_w_tilt_vec)
%%%% 计算平滑递增函数
iiuav = 4;
theta_sigma_bar_w_tilt_1_4 = sigma_bar_w_tilt_squ_1_4(:) .* ( -1 + 2 ./ ( 1 + exp( -alfa_theta_obs_w .* sigma_bar_w_tilt_vec(:,iiuav) ) ) );
theta_sigma_bar_w_tilt_2_4 = sigma_bar_w_tilt_squ_2_4(:) .* ( -1 + 2 ./ ( 1 + exp( -alfa_theta_obs_w .* sigma_bar_w_tilt_vec(:,iiuav) ) ) );

== matlab function sim_tcyb_2024_att_ctrl/cal theta_sigma_bar_w_tilt agent 5 ==
  data: alfa_theta_obs_w input; sigma_bar_w_tilt_squ_1_5 input; theta_sigma_bar_w_tilt_1_5 output; sigma_bar_w_tilt_squ_2_5 input; sigma_bar_w_tilt_vec input; theta_sigma_bar_w_tilt_2_5 output
function [theta_sigma_bar_w_tilt_1_5, theta_sigma_bar_w_tilt_2_5] = fcn(alfa_theta_obs_w, sigma_bar_w_tilt_squ_1_5, sigma_bar_w_tilt_squ_2_5, sigma_bar_w_tilt_vec)
%%%% 计算平滑递增函数
iiuav = 5;
theta_sigma_bar_w_tilt_1_5 = sigma_bar_w_tilt_squ_1_5(:) .* ( -1 + 2 ./ ( 1 + exp( -alfa_theta_obs_w .* sigma_bar_w_tilt_vec(:,iiuav) ) ) );
theta_sigma_bar_w_tilt_2_5 = sigma_bar_w_tilt_squ_2_5(:) .* ( -1 + 2 ./ ( 1 + exp( -alfa_theta_obs_w .* sigma_bar_w_tilt_vec(:,iiuav) ) ) );

== matlab function sim_tcyb_2024_att_ctrl/choose ksi_est_err 11 ==
  data: x input; y output
function y = fcn(x)
iiuav = 1;
y = x(:,iiuav);

== matlab function sim_tcyb_2024_att_ctrl/choose ksi_est_err 12 ==
  data: x input; y output
function y = fcn(x)
iiuav = 1;
y = x(:,iiuav);

== matlab function sim_tcyb_2024_att_ctrl/choose ksi_est_err 13 ==
  data: x input; y output
function y = fcn(x)
iiuav = 2;
y = x(:,iiuav);

== matlab function sim_tcyb_2024_att_ctrl/choose ksi_est_err 14 ==
  data: x input; y output
function y = fcn(x)
iiuav = 2;
y = x(:,iiuav);

== matlab function sim_tcyb_2024_att_ctrl/choose ksi_est_err 15 ==
  data: x input; y output
function y = fcn(x)
iiuav = 3;
y = x(:,iiuav);

== matlab function sim_tcyb_2024_att_ctrl/choose ksi_est_err 16 ==
  data: x input; y output
function y = fcn(x)
iiuav = 3;
y = x(:,iiuav);

== matlab function sim_tcyb_2024_att_ctrl/sgi dynam agent 5 ==
  data: E_sgi_vec input; dsgi_5 output; wi_vec input
function dsgi_5 = fcn(E_sgi_vec, wi_vec)
%%%% 更新四元数微分方程
iiuav = 5;
dsgi_5 = E_sgi_vec(:,:,iiuav) * wi_vec(:,iiuav);
end

== matlab function sim_tcyb_2024_att_ctrl/choose ksi_est_err 17 ==
  data: x input; y output
function y = fcn(x)
iiuav = 4;
y = x(:,iiuav);

== matlab function sim_tcyb_2024_att_ctrl/choose ksi_est_err 18 ==
  data: x input; y output
function y = fcn(x)
iiuav = 4;
y = x(:,iiuav);

== matlab function sim_tcyb_2024_att_ctrl/choose ksi_est_err 19 ==
  data: x input; y output
function y = fcn(x)
iiuav = 5;
y = x(:,iiuav);

== matlab function sim_tcyb_2024_att_ctrl/choose ksi_est_err 20 ==
  data: x input; y output
function y = fcn(x)
iiuav = 5;
y = x(:,iiuav);

== matlab function sim_tcyb_2024_att_ctrl/combine d_sigma_bar_v_est ==
  data: d_sigma_bar_w_est_1 input; d_sigma_bar_w_est_2 input; d_sigma_bar_w_est_3 input; d_sigma_bar_w_est_4 input; d_sigma_bar_w_est_5 input; d_sigma_bar_w_vec output
function d_sigma_bar_w_vec  = fcn(d_sigma_bar_w_est_1, d_sigma_bar_w_est_2, d_sigma_bar_w_est_3, d_sigma_bar_w_est_4, d_sigma_bar_w_est_5)
%%%% 合并用微分器求得的虚拟速度控制量导数
d_sigma_bar_w_vec = [d_sigma_bar_w_est_1(:), d_sigma_bar_w_est_2(:), d_sigma_bar_w_est_3(:), d_sigma_bar_w_est_4(:), d_sigma_bar_w_est_5(:)];

== matlab function sim_tcyb_2024_att_ctrl/combine dw_hat ==
  data: dw_hat_1 input; dw_hat_2 input; dw_hat_3 input; dw_hat_4 input; dw_hat_5 input; dw_hat_vec output
function dw_hat_vec  = fcn(dw_hat_1, dw_hat_2, dw_hat_3, dw_hat_4, dw_hat_5)
%%%% 合并扰动观测值dw_hat
dw_hat_vec = [dw_hat_1(:), dw_hat_2(:), dw_hat_3(:), dw_hat_4(:), dw_hat_5(:)];

== matlab function sim_tcyb_2024_att_ctrl/combine sigma_bar_w_hat ==
  data: sigma_bar_w_hat_1 input; sigma_bar_w_hat_2 input; sigma_bar_w_hat_3 input; sigma_bar_w_hat_4 input; sigma_bar_w_hat_5 input; sigma_bar_w_hat_vec output
function sigma_bar_w_hat_vec  = fcn(sigma_bar_w_hat_1, sigma_bar_w_hat_2, sigma_bar_w_hat_3, sigma_bar_w_hat_4, sigma_bar_w_hat_5)
%%%% 合并虚拟速度控制量观测值sigma_bar_w_hat
sigma_bar_w_hat_vec = [sigma_bar_w_hat_1(:), sigma_bar_w_hat_2(:), sigma_bar_w_hat_3(:), sigma_bar_w_hat_4(:), sigma_bar_w_hat_5(:)];

== matlab function sim_tcyb_2024_att_ctrl/combine sigma_w ==
  data: sigma_w_1 input; sigma_w_vec output; sigma_w_2 input; sigma_w_3 input; sigma_w_4 input; sigma_w_5 input
function sigma_w_vec = fcn(sigma_w_1, sigma_w_2, sigma_w_3, sigma_w_4, sigma_w_5)
%%%% 合并辅助姿态角速率
sigma_w_vec = [sigma_w_1(:), sigma_w_2(:), sigma_w_3(:), sigma_w_4(:), sigma_w_5(:)];

== matlab function sim_tcyb_2024_att_ctrl/combine theta_sigma_bar_w_tilt ==
  data: theta_sigma_bar_w_tilt_1_1 input; theta_sigma_bar_w_tilt_1_2 input; theta_sigma_bar_w_tilt_1_3 input; theta_sigma_bar_w_tilt_1_4 input; theta_sigma_bar_w_tilt_1_5 input; theta_sigma_bar_w_tilt_1_vec output; theta_sigma_bar_w_tilt_2_1 input; theta_sigma_bar_w_tilt_2_vec output; theta_sigma_bar_w_tilt_2_2 input; theta_sigma_bar_w_tilt_2_3 input; theta_sigma_bar_w_tilt_2_4 input; theta_sigma_bar_w_tilt_2_5 input
function [theta_sigma_bar_w_tilt_1_vec, theta_sigma_bar_w_tilt_2_vec]  = fcn(theta_sigma_bar_w_tilt_1_1, theta_sigma_bar_w_tilt_1_2, theta_sigma_bar_w_tilt_1_3, theta_sigma_bar_w_tilt_1_4, theta_sigma_bar_w_tilt_1_5, ...
                                                                                                                                            theta_sigma_bar_w_tilt_2_1, theta_sigma_bar_w_tilt_2_2, theta_sigma_bar_w_tilt_2_3, theta_sigma_bar_w_tilt_2_4, theta_sigma_bar_w_tilt_2_5)
%%%% 合并领导者位置观测器输出结果
theta_sigma_bar_w_tilt_1_vec = [theta_sigma_bar_w_tilt_1_1(:), theta_sigma_bar_w_tilt_1_2(:), theta_sigma_bar_w_tilt_1_3(:), theta_sigma_bar_w_tilt_1_4(:), theta_sigma_bar_w_tilt_1_5(:)];
theta_sigma_bar_w_tilt_2_vec = [theta_sigma_bar_w_tilt_2_1(:), theta_sigma_bar_w_tilt_2_2(:), theta_sigma_bar_w_tilt_2_3(:), theta_sigma_bar_w_tilt_2_4(:), theta_sigma_bar_w_tilt_2_5(:)];

== matlab function sim_tcyb_2024_att_ctrl/dsgei dynam agent 2 ==
  data: E_sgei_vec input; dsgei_2 output; wei_vec input
function dsgei_2 = fcn(E_sgei_vec, wei_vec)
%%%% 更新四元数误差微分方程
iiuav = 2;
dsgei_2 = E_sgei_vec(:,:,iiuav) * wei_vec(:,iiuav);
end

== matlab function sim_tcyb_2024_att_ctrl/trans to column51 ==
  data: x input; y output
function y = fcn(x)
y = x(:);

== matlab function sim_tcyb_2024_att_ctrl/trans to column52 ==
  data: x input; y output
function y = fcn(x)
y = x(:);

== matlab function sim_tcyb_2024_att_ctrl/trans to column53 ==
  data: x input; y output
function y = fcn(x)
y = x(:);

== matlab function sim_tcyb_2024_att_ctrl/trans to column54 ==
  data: x input; y output
function y = fcn(x)
y = x(:);

== matlab function sim_tcyb_2024_att_ctrl/trans to column55 ==
  data: x input; y output
function y = fcn(x)
y = x(:);

== matlab function sim_tcyb_2024_att_ctrl/trans to column56 ==
  data: x input; y output
function y = fcn(x)
y = x(:);

== matlab function sim_tcyb_2024_att_ctrl/trans to column57 ==
  data: x input; y output
function y = fcn(x)
y = x(:);

== matlab function sim_tcyb_2024_att_ctrl/trans to column58 ==
  data: x input; y output
function y = fcn(x)
y = x(:);

== matlab function sim_tcyb_2024_att_ctrl/trans to column59 ==
  data: x input; y output
function y = fcn(x)
y = x(:);

== matlab function sim_tcyb_2024_att_ctrl/trans to column60 ==
  data: x input; y output
function y = fcn(x)
y = x(:);

== matlab function sim_tcyb_2024_att_ctrl/E_sgei agent 3 ==
  data: sgei_vec input; E_sgei_3 output
function E_sgei_3 = fcn(sgei_vec)
%%%% 更新四元数微分方程
iiuav = 3;
E_sgei_3 = (1/4) * ( ( 1 - (sgei_vec(:,iiuav)') * sgei_vec(:,iiuav) ) * eye(3) ...
                    + 2 * cal_askew_mat( sgei_vec(:,iiuav) ) + 2 * sgei_vec(:,iiuav) * ( sgei_vec(:,iiuav)' ) );
end

== matlab function sim_tcyb_2024_att_ctrl/combine tau1 ==
  data: dw_1 input; dw_vec output; dw_2 input; dw_3 input; dw_4 input; dw_5 input
function dw_vec = fcn(dw_1, dw_2, dw_3, dw_4, dw_5)
%%%% 合并辅助姿态角速率
dw_vec = [dw_1(:), dw_2(:), dw_3(:), dw_4(:), dw_5(:)];

== matlab function sim_tcyb_2024_att_ctrl/generate angular rate disturbance agent 1 ==
  data: dw_1 output; dw_aa_t input; dw_ff_t input; dw_phi_t input; t input
function dw_1 = fcn(dw_aa_t, dw_ff_t, dw_phi_t, t)
%%%% 姿态动力学方程中的扰动项设置
epsil_t = zeros(3, 1);

for kk = 1:5
    epsil_t = epsil_t + dw_aa_t(:, kk) .* sin( 2 * pi * dw_ff_t(:, kk) * t + dw_phi_t(:, kk) );
end

dw_1 = [ epsil_t(1) + 1.6 * sin( 0.4 * t ) + 2.0 * cos( 0.5 * t ) + 1.4 * sin( 0.7 * t ) ...
                + 4 * exp( -0.1 * t ) * sin( 0.8 * t ) + 3 / ( 1 + exp( -0.2 * ( t - 15 ) ) ); ...
                epsil_t(2) + 1.2 * sin( 0.2 * t ) + 3 * cos( 0.4 * t ) + 0.8 * sin( 0.6 * t ) ...
                + 2 * exp( -0.15 * t ) * cos( 1.2 * t ) + 3 / ( 1 + exp( -0.3 * ( t - 25 ) ) ); ...
                epsil_t(3) + 1.8 * sin( 0.2 * t ) + 1.6 * sin( 0.3 * t ) + 1.6 * cos( 0.4 * t ) ...
                + 4 * exp( -0.05 * t ) * sin( 0.5 * t + pi / 4 ) + 3 / ( 1 + exp( -0.5 * ( t - 20 ) ) ) ];

== matlab function sim_tcyb_2024_att_ctrl/generate angular rate disturbance agent 2 ==
  data: dw_2 output; dw_aa_t input; dw_ff_t input; dw_phi_t input; t input
function dw_2 = fcn(dw_aa_t, dw_ff_t, dw_phi_t, t)
%%%% 姿态动力学方程中的扰动项设置
epsil_t = zeros(3, 1);

for kk = 1:5
    epsil_t = epsil_t + dw_aa_t(:, kk) .* sin( 2 * pi * dw_ff_t(:, kk) * t + dw_phi_t(:, kk) );
end

dw_2 = [ epsil_t(1) + 1.6 * sin( 0.2 * t ) + 2.0 * cos( 0.3 * t ) + 1.4 * sin( 0.5 * t ) ...
                + 4 * exp( -0.1 * t ) * sin( 0.5 * t ) + 3 / ( 1 + exp( -0.2 * ( t - 15 ) ) ); ...
                epsil_t(2) + 1.2 * sin( 0.1 * t ) + 3 * cos( 0.2 * t ) + 0.8 * sin( 0.4 * t ) ...
                + 2 * exp( -0.15 * t ) * cos( 0.6 * t ) + 3 / ( 1 + exp( -0.3 * ( t - 25 ) ) ); ...
                epsil_t(3) + 1.8 * sin( 0.1 * t ) + 1.6 * sin( 0.2 * t ) + 1.6 * cos( 0.3 * t ) ...
                + 4 * exp( -0.05 * t ) * sin( 0.4 * t + pi / 4 ) + 3 / ( 1 + exp( -0.5 * ( t - 20 ) ) ) ];

== matlab function sim_tcyb_2024_att_ctrl/generate angular rate disturbance agent 3 ==
  data: dw_3 output; dw_aa_t input; dw_ff_t input; dw_phi_t input; t input
function dw_3 = fcn(dw_aa_t, dw_ff_t, dw_phi_t, t)
%%%% 姿态动力学方程中的扰动项设置
epsil_t = zeros(3, 1);

for kk = 1:5
    epsil_t = epsil_t + dw_aa_t(:, kk) .* sin( 2 * pi * dw_ff_t(:, kk) * t + dw_phi_t(:, kk) );
end

dw_3 = [ epsil_t(1) + 1.6 * sin( 0.2 * t ) + 2.0 * cos( 0.3 * t ) + 1.4 * sin( 0.5 * t ) ...
                + 4 * exp( -0.1 * t ) * sin( 0.5 * t ) + 3 / ( 1 + exp( -0.2 * ( t - 15 ) ) ); ...
                epsil_t(2) + 1.2 * sin( 0.1 * t ) + 3 * cos( 0.2 * t ) + 0.8 * sin( 0.4 * t ) ...
                + 2 * exp( -0.15 * t ) * cos( 0.6 * t ) + 3 / ( 1 + exp( -0.3 * ( t - 25 ) ) ); ...
                epsil_t(3) + 1.8 * sin( 0.1 * t ) + 1.6 * sin( 0.2 * t ) + 1.6 * cos( 0.3 * t ) ...
                + 4 * exp( -0.05 * t ) * sin( 0.4 * t + pi / 4 ) + 3 / ( 1 + exp( -0.5 * ( t - 20 ) ) ) ];

== matlab function sim_tcyb_2024_att_ctrl/generate angular rate disturbance agent 4 ==
  data: dw_4 output; dw_aa_t input; dw_ff_t input; dw_phi_t input; t input
function dw_4 = fcn(dw_aa_t, dw_ff_t, dw_phi_t, t)
%%%% 姿态动力学方程中的扰动项设置
epsil_t = zeros(3, 1);

for kk = 1:5
    epsil_t = epsil_t + dw_aa_t(:, kk) .* sin( 2 * pi * dw_ff_t(:, kk) * t + dw_phi_t(:, kk) );
end

dw_4 = [ epsil_t(1) + 1.6 * sin( 0.2 * t ) + 2.0 * cos( 0.3 * t ) + 1.4 * sin( 0.5 * t ) ...
                + 4 * exp( -0.1 * t ) * sin( 0.5 * t ) + 3 / ( 1 + exp( -0.2 * ( t - 15 ) ) ); ...
                epsil_t(2) + 1.2 * sin( 0.1 * t ) + 3 * cos( 0.2 * t ) + 0.8 * sin( 0.4 * t ) ...
                + 2 * exp( -0.15 * t ) * cos( 0.6 * t ) + 3 / ( 1 + exp( -0.3 * ( t - 25 ) ) ); ...
                epsil_t(3) + 1.8 * sin( 0.1 * t ) + 1.6 * sin( 0.2 * t ) + 1.6 * cos( 0.3 * t ) ...
                + 4 * exp( -0.05 * t ) * sin( 0.4 * t + pi / 4 ) + 3 / ( 1 + exp( -0.5 * ( t - 20 ) ) ) ];

== matlab function sim_tcyb_2024_att_ctrl/generate angular rate disturbance agent 5 ==
  data: dw_5 output; dw_aa_t input; dw_ff_t input; dw_phi_t input; t input
function dw_5 = fcn(dw_aa_t, dw_ff_t, dw_phi_t, t)
%%%% 姿态动力学方程中的扰动项设置
epsil_t = zeros(3, 1);

for kk = 1:5
    epsil_t = epsil_t + dw_aa_t(:, kk) .* sin( 2 * pi * dw_ff_t(:, kk) * t + dw_phi_t(:, kk) );
end

dw_5 = [ epsil_t(1) + 1.6 * sin( 0.2 * t ) + 2.0 * cos( 0.3 * t ) + 1.4 * sin( 0.5 * t ) ...
                + 4 * exp( -0.1 * t ) * sin( 0.5 * t ) + 3 / ( 1 + exp( -0.2 * ( t - 15 ) ) ); ...
                epsil_t(2) + 1.2 * sin( 0.1 * t ) + 3 * cos( 0.2 * t ) + 0.8 * sin( 0.4 * t ) ...
                + 2 * exp( -0.15 * t ) * cos( 0.6 * t ) + 3 / ( 1 + exp( -0.3 * ( t - 25 ) ) ); ...
                epsil_t(3) + 1.8 * sin( 0.1 * t ) + 1.6 * sin( 0.2 * t ) + 1.6 * cos( 0.3 * t ) ...
                + 4 * exp( -0.05 * t ) * sin( 0.4 * t + pi / 4 ) + 3 / ( 1 + exp( -0.5 * ( t - 20 ) ) ) ];

== matlab function sim_tcyb_2024_att_ctrl/combine norminal formation control input ==
  data: ui_1 input; ui_vec output; ui_2 input; ui_3 input; ui_4 input; ui_5 input
function ui_vec = fcn(ui_1, ui_2, ui_3, ui_4, ui_5)
%%%% 合并领导者编队跟踪误差结果
ui_vec = [ui_1(:), ui_2(:), ui_3(:), ui_4(:), ui_5(:)];

== matlab function sim_tcyb_2024_att_ctrl/cal Rei agent 3 ==
  data: Rei_3 output; sgei_vec input
function Rei_3 = fcn(sgei_vec)
%%%% 由罗德里格常量sgi求解姿态旋转矩阵Ri
iiuav = 3;
Rei_3 = eye(3) + 4 * ( 1 - ( ( ( sgei_vec(:,iiuav)' ) * sgei_vec(:,iiuav) ) / ( ( 1 + ( sgei_vec(:,iiuav)' ) * sgei_vec(:,iiuav) ) ^ 2 ) ) ) * cal_askew_mat( sgei_vec(:,iiuav) ) ...
                            + ( 8 / ( ( 1 + ( sgei_vec(:,iiuav)' ) * sgei_vec(:,iiuav) ) ^ 2 ) ) * cal_askew_mat( sgei_vec(:,iiuav) ) * cal_askew_mat( sgei_vec(:,iiuav) );
Rei_3 = Rei_3';
end

== matlab function sim_tcyb_2024_att_ctrl/control input generator agent 1 ==
  data: u0 input; ui output
function ui  = fcn(u0)
%%%% 给出领导者参考加速度控制输入
g0 = 9.80663;
e3 = [0;0;1];

ui = g0 * e3 + u0(:);

== matlab function sim_tcyb_2024_att_ctrl/control input generator agent 2 ==
  data: u0 input; ui output
function ui  = fcn(u0)
%%%% 给出领导者参考加速度控制输入
g0 = 9.80663;
e3 = [0;0;1];

ui = g0 * e3 + u0(:);

== matlab function sim_tcyb_2024_att_ctrl/control input generator agent 3 ==
  data: u0 input; ui output
function ui  = fcn(u0)
%%%% 给出领导者参考加速度控制输入
g0 = 9.80663;
e3 = [0;0;1];

ui = g0 * e3 + u0(:);

== matlab function sim_tcyb_2024_att_ctrl/control input generator agent 4 ==
  data: u0 input; ui output
function ui  = fcn(u0)
%%%% 给出领导者参考加速度控制输入
g0 = 9.80663;
e3 = [0;0;1];

ui = g0 * e3 + u0(:);

== matlab function sim_tcyb_2024_att_ctrl/control input generator agent 5 ==
  data: u0 input; ui output
function ui  = fcn(u0)
%%%% 给出领导者参考加速度控制输入
g0 = 9.80663;
e3 = [0;0;1];

ui = g0 * e3 + u0(:);

== matlab function sim_tcyb_2024_att_ctrl/cal wei agent 3 ==
  data: wi_vec input; wei_3 output; Rei_vec input; wci_vec input
function wei_3 = fcn(wi_vec, Rei_vec, wci_vec)
%%%% 更新姿态角速率误差
iiuav = 3;
wei_3 = wi_vec(:,iiuav) - (Rei_vec(:,:,iiuav)') * wci_vec(:,iiuav);
end

== matlab function sim_tcyb_2024_att_ctrl/dsgei dynam agent 3 ==
  data: E_sgei_vec input; dsgei_3 output; wei_vec input
function dsgei_3 = fcn(E_sgei_vec, wei_vec)
%%%% 更新四元数误差微分方程
iiuav = 3;
dsgei_3 = E_sgei_vec(:,:,iiuav) * wei_vec(:,iiuav);
end

== matlab function sim_tcyb_2024_att_ctrl/E_sgei agent 4 ==
  data: sgei_vec input; E_sgei_4 output
function E_sgei_4 = fcn(sgei_vec)
%%%% 更新四元数微分方程
iiuav = 4;
E_sgei_4 = (1/4) * ( ( 1 - (sgei_vec(:,iiuav)') * sgei_vec(:,iiuav) ) * eye(3) ...
                    + 2 * cal_askew_mat( sgei_vec(:,iiuav) ) + 2 * sgei_vec(:,iiuav) * ( sgei_vec(:,iiuav)' ) );
end

== matlab function sim_tcyb_2024_att_ctrl/cal Rei agent 4 ==
  data: Rei_4 output; sgei_vec input
function Rei_4 = fcn(sgei_vec)
%%%% 由罗德里格常量sgi求解姿态旋转矩阵Ri
iiuav = 4;
Rei_4 = eye(3) + 4 * ( 1 - ( ( ( sgei_vec(:,iiuav)' ) * sgei_vec(:,iiuav) ) / ( ( 1 + ( sgei_vec(:,iiuav)' ) * sgei_vec(:,iiuav) ) ^ 2 ) ) ) * cal_askew_mat( sgei_vec(:,iiuav) ) ...
                            + ( 8 / ( ( 1 + ( sgei_vec(:,iiuav)' ) * sgei_vec(:,iiuav) ) ^ 2 ) ) * cal_askew_mat( sgei_vec(:,iiuav) ) * cal_askew_mat( sgei_vec(:,iiuav) );
Rei_4 = Rei_4';
end

== matlab function sim_tcyb_2024_att_ctrl/cal wei agent 4 ==
  data: wi_vec input; wei_4 output; Rei_vec input; wci_vec input
function wei_4 = fcn(wi_vec, Rei_vec, wci_vec)
%%%% 更新姿态角速率误差
iiuav = 4;
wei_4 = wi_vec(:,iiuav) - (Rei_vec(:,:,iiuav)') * wci_vec(:,iiuav);
end

== matlab function sim_tcyb_2024_att_ctrl/dsgei dynam agent 4 ==
  data: E_sgei_vec input; dsgei_4 output; wei_vec input
function dsgei_4 = fcn(E_sgei_vec, wei_vec)
%%%% 更新四元数误差微分方程
iiuav = 4;
dsgei_4 = E_sgei_vec(:,:,iiuav) * wei_vec(:,iiuav);
end

== matlab function sim_tcyb_2024_att_ctrl/cal d_theta_hat ==
  data: c1 input; d_ui_hat output; d_dui_hat output; d_d2ui_hat output; c2 input; c3 input; chi_t input; ui_sig_1 input; ui_sig_2 input; ui_sig_3 input; ui_sig_4 input; ui_sig_5 input; ui_sig_6 input; dui_hat input; d2ui_hat input
function [d_ui_hat, d_dui_hat, d_d2ui_hat] = fcn(c1, c2, c3, chi_t, ui_sig_1, ui_sig_2, ui_sig_3, ...
                                                                                        ui_sig_4, ui_sig_5, ui_sig_6, dui_hat, d2ui_hat)
d_d2ui_hat = -chi_t .* c1 * ui_sig_1(:) - (1 - chi_t) .* c1 * ui_sig_2(:);
d_dui_hat = -chi_t .* c2 * ui_sig_3(:) - (1 - chi_t) .* c2 * ui_sig_4(:) + d2ui_hat(:);
d_ui_hat = -chi_t .* c3 * ui_sig_5(:) - (1 - chi_t) .* c3 * ui_sig_6(:) + dui_hat(:);

== matlab function sim_tcyb_2024_att_ctrl/E_sgei agent 5 ==
  data: sgei_vec input; E_sgei_5 output
function E_sgei_5 = fcn(sgei_vec)
%%%% 更新四元数微分方程
iiuav = 5;
E_sgei_5 = (1/4) * ( ( 1 - (sgei_vec(:,iiuav)') * sgei_vec(:,iiuav) ) * eye(3) ...
                    + 2 * cal_askew_mat( sgei_vec(:,iiuav) ) + 2 * sgei_vec(:,iiuav) * ( sgei_vec(:,iiuav)' ) );
end

== matlab function sim_tcyb_2024_att_ctrl/cal Rei agent 5 ==
  data: Rei_5 output; sgei_vec input
function Rei_5 = fcn(sgei_vec)
%%%% 由罗德里格常量sgi求解姿态旋转矩阵Ri
iiuav = 5;
Rei_5 = eye(3) + 4 * ( 1 - ( ( ( sgei_vec(:,iiuav)' ) * sgei_vec(:,iiuav) ) / ( ( 1 + ( sgei_vec(:,iiuav)' ) * sgei_vec(:,iiuav) ) ^ 2 ) ) ) * cal_askew_mat( sgei_vec(:,iiuav) ) ...
                            + ( 8 / ( ( 1 + ( sgei_vec(:,iiuav)' ) * sgei_vec(:,iiuav) ) ^ 2 ) ) * cal_askew_mat( sgei_vec(:,iiuav) ) * cal_askew_mat( sgei_vec(:,iiuav) );
Rei_5 = Rei_5';
end

== matlab function sim_tcyb_2024_att_ctrl/cal wei agent 5 ==
  data: wi_vec input; wei_5 output; Rei_vec input; wci_vec input
function wei_5 = fcn(wi_vec, Rei_vec, wci_vec)
%%%% 更新姿态角速率误差
iiuav = 5;
wei_5 = wi_vec(:,iiuav) - (Rei_vec(:,:,iiuav)') * wci_vec(:,iiuav);
end

== matlab function sim_tcyb_2024_att_ctrl/dsgei dynam agent 5 ==
  data: E_sgei_vec input; dsgei_5 output; wei_vec input
function dsgei_5 = fcn(E_sgei_vec, wei_vec)
%%%% 更新四元数误差微分方程
iiuav = 5;
dsgei_5 = E_sgei_vec(:,:,iiuav) * wei_vec(:,iiuav);
end

== matlab function sim_tcyb_2024_att_ctrl/combine E_sgi_vec1 ==
  data: E_sgei_1 input; E_sgei_vec output; E_sgei_2 input; E_sgei_3 input; E_sgei_4 input; E_sgei_5 input
function E_sgei_vec = fcn(E_sgei_1, E_sgei_2, E_sgei_3, E_sgei_4, E_sgei_5)
%%%% 合并姿态计算矩阵
E_sgei_vec = zeros(3,3,5);
E_sgei_vec(:,:,1) = E_sgei_1;
E_sgei_vec(:,:,2) = E_sgei_2;
E_sgei_vec(:,:,3) = E_sgei_3;
E_sgei_vec(:,:,4) = E_sgei_4;
E_sgei_vec(:,:,5) = E_sgei_5;

== matlab function sim_tcyb_2024_att_ctrl/cal Gamma_wi agent 1 ==
  data: wi_vec input; Gamma_wi_1 output
function Gamma_wi_1 = fcn(wi_vec)
%%%% 计算矩阵 Gamma_wi
iiuav = 1;
Gamma_wi_1 = [wi_vec(1,iiuav), 0, 0, 0, wi_vec(3,iiuav), wi_vec(2,iiuav); ...
                                0, wi_vec(2,iiuav), 0, wi_vec(3,iiuav), 0, wi_vec(1,iiuav); ...
                                0, 0, wi_vec(3,iiuav), wi_vec(2,iiuav), wi_vec(1,iiuav), 0];
end

== matlab function sim_tcyb_2024_att_ctrl/cal sig ==
  data: x input; z output; y input
function z = fcn(x, y)
z = x(:) .* sign(y(:));

== matlab function sim_tcyb_2024_att_ctrl/cal sig1 ==
  data: x input; z output; y input
function z = fcn(x, y)
z = x(:) .* sign(y(:));

== matlab function sim_tcyb_2024_att_ctrl/cal sig2 ==
  data: x input; z output; y input
function z = fcn(x, y)
z = x(:) .* sign(y(:));

== matlab function sim_tcyb_2024_att_ctrl/cal sig3 ==
  data: x input; z output; y input
function z = fcn(x, y)
z = x(:) .* sign(y(:));

== matlab function sim_tcyb_2024_att_ctrl/cal sig4 ==
  data: x input; z output; y input
function z = fcn(x, y)
z = x(:) .* sign(y(:));

== matlab function sim_tcyb_2024_att_ctrl/cal sig5 ==
  data: x input; z output; y input
function z = fcn(x, y)
z = x(:) .* sign(y(:));

== matlab function sim_tcyb_2024_att_ctrl/trans to column10 ==
  data: x input; y output
function y = fcn(x)
y = x(:);

== matlab function sim_tcyb_2024_att_ctrl/trans to column5 ==
  data: x input; y output
function y = fcn(x)
y = x(:);

== matlab function sim_tcyb_2024_att_ctrl/trans to column6 ==
  data: x input; y output
function y = fcn(x)
y = x(:);

== matlab function sim_tcyb_2024_att_ctrl/trans to column7 ==
  data: x input; y output
function y = fcn(x)
y = x(:);

== matlab function sim_tcyb_2024_att_ctrl/trans to column8 ==
  data: x input; y output
function y = fcn(x)
y = x(:);

== matlab function sim_tcyb_2024_att_ctrl/trans to column9 ==
  data: x input; y output
function y = fcn(x)
y = x(:);

== matlab function sim_tcyb_2024_att_ctrl/choose ui agent 1 ==
  data: x input; y output
function y = fcn(x)
iiuav = 1;
y = x(:,iiuav);

== matlab function sim_tcyb_2024_att_ctrl/cal d_theta_hat1 ==
  data: c1 input; d_ui_hat output; d_dui_hat output; d_d2ui_hat output; c2 input; c3 input; chi_t input; ui_sig_1 input; ui_sig_2 input; ui_sig_3 input; ui_sig_4 input; ui_sig_5 input; ui_sig_6 input; dui_hat input; d2ui_hat input
function [d_ui_hat, d_dui_hat, d_d2ui_hat] = fcn(c1, c2, c3, chi_t, ui_sig_1, ui_sig_2, ui_sig_3, ...
                                                                                        ui_sig_4, ui_sig_5, ui_sig_6, dui_hat, d2ui_hat)
d_d2ui_hat = -chi_t .* c1 * ui_sig_1(:) - (1 - chi_t) .* c1 * ui_sig_2(:);
d_dui_hat = -chi_t .* c2 * ui_sig_3(:) - (1 - chi_t) .* c2 * ui_sig_4(:) + d2ui_hat(:);
d_ui_hat = -chi_t .* c3 * ui_sig_5(:) - (1 - chi_t) .* c3 * ui_sig_6(:) + dui_hat(:);

== matlab function sim_tcyb_2024_att_ctrl/cal sig10 ==
  data: x input; z output; y input
function z = fcn(x, y)
z = x(:) .* sign(y(:));

== matlab function sim_tcyb_2024_att_ctrl/cal sig11 ==
  data: x input; z output; y input
function z = fcn(x, y)
z = x(:) .* sign(y(:));

== matlab function sim_tcyb_2024_att_ctrl/cal sig6 ==
  data: x input; z output; y input
function z = fcn(x, y)
z = x(:) .* sign(y(:));

== matlab function sim_tcyb_2024_att_ctrl/cal sig7 ==
  data: x input; z output; y input
function z = fcn(x, y)
z = x(:) .* sign(y(:));

== matlab function sim_tcyb_2024_att_ctrl/cal sig8 ==
  data: x input; z output; y input
function z = fcn(x, y)
z = x(:) .* sign(y(:));

== matlab function sim_tcyb_2024_att_ctrl/cal sig9 ==
  data: x input; z output; y input
function z = fcn(x, y)
z = x(:) .* sign(y(:));

== matlab function sim_tcyb_2024_att_ctrl/choose ui agent 2 ==
  data: x input; y output
function y = fcn(x)
iiuav = 2;
y = x(:,iiuav);

== matlab function sim_tcyb_2024_att_ctrl/trans to column11 ==
  data: x input; y output
function y = fcn(x)
y = x(:);

== matlab function sim_tcyb_2024_att_ctrl/trans to column12 ==
  data: x input; y output
function y = fcn(x)
y = x(:);

== matlab function sim_tcyb_2024_att_ctrl/trans to column13 ==
  data: x input; y output
function y = fcn(x)
y = x(:);

== matlab function sim_tcyb_2024_att_ctrl/trans to column14 ==
  data: x input; y output
function y = fcn(x)
y = x(:);

== matlab function sim_tcyb_2024_att_ctrl/trans to column15 ==
  data: x input; y output
function y = fcn(x)
y = x(:);
